simulink model "modelo_lqr_n_linear"  (R2023a)
settings: Solver=ode45  StartTime=0.0  StopTime=10  MaxStep=0.01  RelTol=1e-3
model workspace: external: MATLAB File C:\Users\pinki\OneDrive\aviãozinho\monociclo\numvars.m (data not in the file)
values from neighbouring files (symbols this model uses):
  Ard = [Ar(1,1) Ar(1,3:end) ... (first row only)    [Modelo_mono.m]    (also in workspace.mat = [0 0 -31.2551437046 31.2551437046 0 0 0 0 0 0 -92.3888975157)
  Brd = [Br(1,:) ... (first row only)    [Modelo_mono.m]    (also in workspace.mat = [0  0; 0  0; 50297.8358889  0; -78.116759971  0; 0  238.3657)
  Crd = eye(6)    [Modelo_mono.m]    (also in workspace.mat = [1 0 0 0 0 0 0 1 0 0 0 0 ... (36 elements, 6x6)])
  Jbw = 0.07689    [Modelo_mono.m]    (also in gab_numvars.m; modelo.mat; numvars.m; workspace.mat = 0.026534412)
  Jr = 0.013472    [Modelo_mono.m]    (also in gab_numvars.m; modelo.mat; numvars.m; workspace.mat = 0.0001347355)
  K = lqr(Ard,Brd,Qc,Rc)    [Modelo_mono.m]    (also in cascatinha_v3.m = [tprK,0; workspace.mat = [-891.058429104  -1.00065730536e-12  -0.217264538579  -159.5)
  v_ic = [0;0;0;0]    [Modelo_mono.m]    (also in workspace.mat = [0 0 0 0])
  x_ic = [0;5*pi/180;0;-5*pi/180]    [Modelo_mono.m]    (also in workspace.mat = [0 0.0872664625997 0 -0.0872664625997])
libraries: simulink_extras x1
settings Model: Creator=pinki  LastModifiedBy=pinki
settings DataIOCC: InspectSignalLogs=on

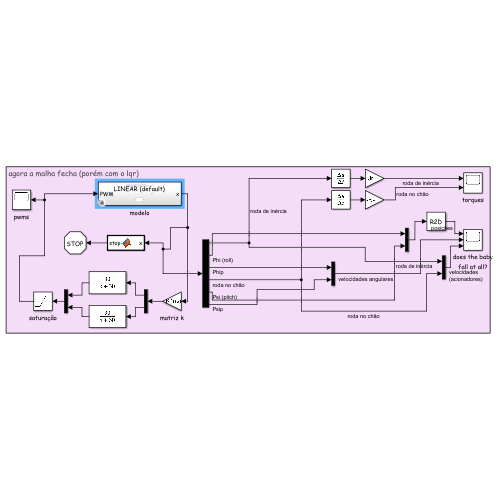
[thumbnail: Simulink's stored preview of the top-level diagram]
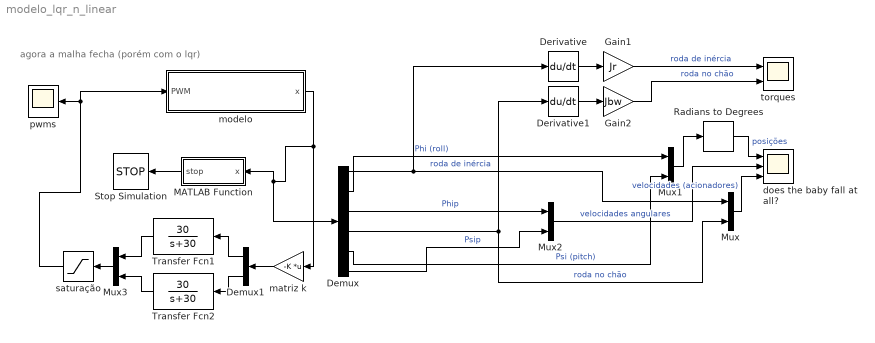
== system modelo_lqr_n_linear ==
  note: agora a malha fecha (porém com o lqr)
  Demux : Demux  Outputs=6
  Demux1 : Demux  Outputs=2
  Derivative : Derivative
  Derivative1 : Derivative
  Gain1 : Gain  Gain=Jr
  Gain2 : Gain  Gain=Jbw
  MATLAB Function : MATLAB Function  TreatAsAtomicUnit=on
  Mux{,1..3} (4 alike) : Mux  Inputs=2
  Radians to Degrees : simulink_extras/Transformations/Radians to Degrees
  Stop Simulation : Stop
  Transfer Fcn1 : TransferFcn  Numerator=[30]  Denominator=[1 30]
  Transfer Fcn2 : TransferFcn  Numerator=[30]  Denominator=[1 30]
  does the baby fall at all? : Scope  NumInputPorts=3
  matriz k : Gain  Gain=-K  Multiplication=Matrix(K*u) (u vector)
  modelo : Subsystem  Variant=on  VariantControlMode=label  LabelModeActiveChoice=(default)
  pwms : Scope
  saturação : Saturate  UpperLimit=1  LowerLimit=-1
  torques : Scope  NumInputPorts=2
  wires:
  modelo/1(x) -> Demux/1, MATLAB Function/1(x), matriz k/1
  Demux/1 -> Derivative/1, Mux/1  "roda de inércia"
  Demux/4 -> Mux/2, Derivative1/1  "roda no chão"
  Demux/3 -> Mux2/1  "Phip"
  saturação/1 -> modelo/1(PWM), pwms/1
  MATLAB Function/1(stop) -> Stop Simulation/1
  Derivative/1 -> Gain1/1
  Gain1/1 -> torques/1  "roda de inércia"
  Derivative1/1 -> Gain2/1
  Gain2/1 -> torques/2  "roda no chão"
  Demux/2 -> Mux1/1  "Phi (roll)"
  Demux/6 -> Mux2/2  "Psip"
  Demux/5 -> Mux1/2  "Psi (pitch)"
  Mux1/1 -> Radians to Degrees/1
  Mux2/1 -> does the baby fall at all?/2  "velocidades angulares"
  Mux/1 -> does the baby fall at all?/3  "velocidades (acionadores)"
  matriz k/1 -> Demux1/1
  Demux1/1 -> Transfer Fcn1/1
  Demux1/2 -> Transfer Fcn2/1
  Transfer Fcn2/1 -> Mux3/2
  Transfer Fcn1/1 -> Mux3/1
  Mux3/1 -> saturação/1
  Radians to Degrees/1 -> does the baby fall at all?/1  "posições"

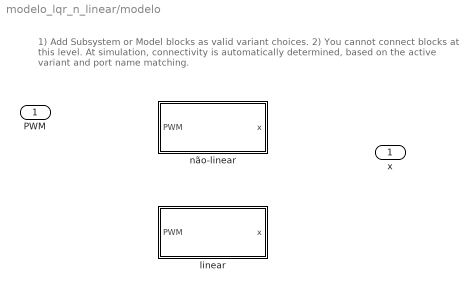
== system modelo_lqr_n_linear/modelo ==
  note: 1) Add Subsystem or Model blocks as valid variant choices.
      | 2) You cannot connect blocks at this level. At simulation, connectivity is automatically
      | determined, based on the active variant and port name matching.
  PWM : Inport
  linear : Subsystem  VariantControl=(default)
  não-linear : Subsystem  VariantControl=nonlinear
  x : Outport

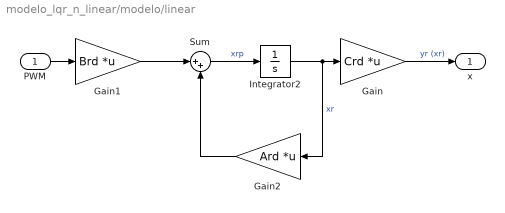
== system modelo_lqr_n_linear/modelo/linear ==
  PWM : Inport
  Gain : Gain  Gain=Crd  Multiplication=Matrix(K*u) (u vector)
  Gain1 : Gain  Gain=Brd  Multiplication=Matrix(K*u) (u vector)
  Gain2 : Gain  Gain=Ard  Multiplication=Matrix(K*u) (u vector)
  Integrator2 : Integrator  InitialCondition=x_ic
  Sum : Sum  Inputs=|++
  x : Outport
  wires:
  PWM/1 -> Gain1/1
  Integrator2/1 -> Gain2/1, Gain/1  "xr"
  Gain/1 -> x/1  "yr (xr)"
  Gain1/1 -> Sum/1
  Sum/1 -> Integrator2/1  "xrp"
  Gain2/1 -> Sum/2

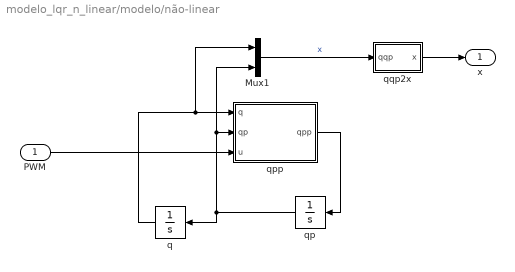
== system modelo_lqr_n_linear/modelo/não-linear ==
  PWM : Inport
  Mux1 : Mux  Inputs=2
  q : Integrator  InitialCondition=x_ic  ContinuousStateAttributes='q'
  qp : Integrator  InitialCondition=v_ic  ContinuousStateAttributes='qp'
  qpp : MATLAB Function  Description=nonlinear model  TreatAsAtomicUnit=on
  qqp2x : Subsystem
  x : Outport
  wires:
  qp/1 -> Mux1/2, qpp/2(qp), q/1
  PWM/1 -> qpp/3(u)
  Mux1/1 -> qqp2x/1(qqp)  "x"
  q/1 -> Mux1/1, qpp/1(q)
  qpp/1(qpp) -> qp/1
  qqp2x/1(x) -> x/1

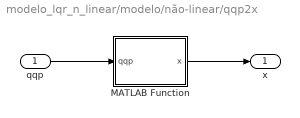
== system modelo_lqr_n_linear/modelo/não-linear/qqp2x ==
  qqp : Inport
  MATLAB Function : MATLAB Function  TreatAsAtomicUnit=on
  x : Outport
  wires:
  qqp/1 -> MATLAB Function/1(qqp)
  MATLAB Function/1(x) -> x/1

== matlab function modelo_lqr_n_linear/MATLAB Function ==
  data: x input; stop output
function stop = fcn(x)

Roll = x(2);
Pitch = x(5);

%% assumindo deslocamento m'aximo de 30 graus ou 0,5 rad...
limite = 0.5;

stop = abs(Pitch)>limite || abs(Roll)>limite;

== matlab function modelo_lqr_n_linear/modelo/não-linear/qqp2x/MATLAB Function ==
  data: qqp input; x output
function x = fcn(qqp)

x = [qqp(5);...
     qqp(2);...
     qqp(6);...
     qqp(7);...
     qqp(4);...
     qqp(8)];

== matlab function modelo_lqr_n_linear/modelo/não-linear/qpp ==
  data: q input; qp input; qpp output; u input
function qpp = fun(q,qp,u)

%% setup
mono = monociclo;

phi = q(2);
psi = q(4);

phi_d = qp(2);
psi_d = qp(4);

thetad_d = qp(1);
thetaw_d = qp(3);

%% setup 2: electric boogaloo
M = fM(mono.jbr, mono.jbw, mono.jr, mono.jw, mono.l, mono.mb, mono.mr, mono.mw, mono.rw, mono.d, psi);
N = fN(mono.ker, mono.kew, mono.ktr, mono.ktw, mono.l, mono.mb, mono.mr, mono.rr, mono.rw, mono.rw, mono.d, mono.nr, mono.nw, phi_d, psi, psi_d, thetad_d, thetaw_d);
O = fO(mono.l, mono.mb, mono.mr, mono.mw, mono.rw, mono.d, mono.g, phi, phi);
P = fP(mono.ktr, mono.ktw, mono.rr, mono.rw, mono.nr, mono.nw);

function M = fM(Jbr,Jbw,Jr,Jw,L,Mb,Mr,Mw,Rw,d,psi_)
%    This function was generated by the Symbolic Math Toolbox version 9.3.

t2 = cos(psi_);
t3 = Mr.*d;
t4 = L.^2;
t5 = Rw.^2;
t7 = L.*Mb;
t8 = L.*Mr;
t9 = t2.^2;
t10 = Mb.*t5;
t11 = Mr.*t5;
t12 = Mw.*t5;
t13 = t3+t7+t8;
t14 = Rw.*t2.*t13;
M = reshape([Jr,Jr,0.0,0.0,Jr,Jbw+Jr+t10+t11+t12+L.*t3.*t9.*2.0+Mb.*t4.*t9+Mr.*t4.*t9+Rw.*t2.*t3.*2.0+Rw.*t2.*t7.*2.0+Rw.*t2.*t8.*2.0+d.*t3.*t9,0.0,0.0,0.0,0.0,Jw+t10+t11+t12,t14,0.0,0.0,t14,Jbr+L.*t3.*2.0+Mb.*t4+Mr.*t4+d.*t3],[4,4]);
end

function N = fN(Ke_d,Ke_w,Kt_d,Kt_w,L,Mb,Mr,R_d,R_w,Rw,d,n_d,n_w,phi_d,psi_,psi_d,thetad_d,thetaw_d)
%    This function was generated by the Symbolic Math Toolbox version 9.3.

t2 = sin(psi_);
t3 = L.^2;
t4 = d.^2;
t5 = n_d.^2;
t6 = n_w.^2;
t7 = phi_d.^2;
t8 = psi_.*2.0;
t9 = psi_d.^2;
t11 = 1.0./R_d;
t12 = 1.0./R_w;
t10 = sin(t8);
t13 = Ke_w.*Kt_w.*n_w.*psi_d.*t12;
t14 = Ke_d.*Kt_d.*t5.*t11.*thetad_d;
t15 = Ke_w.*Kt_w.*t6.*t12.*thetaw_d;
N = [t14;-t14-Mb.*phi_d.*psi_d.*t3.*t10-Mr.*phi_d.*psi_d.*t3.*t10-Mr.*phi_d.*psi_d.*t4.*t10-L.*Mb.*Rw.*phi_d.*psi_d.*t2.*2.0-L.*Mr.*Rw.*phi_d.*psi_d.*t2.*2.0-L.*Mr.*d.*phi_d.*psi_d.*t10.*2.0-Mr.*Rw.*d.*phi_d.*psi_d.*t2.*2.0;-t13+t15-L.*Mb.*Rw.*t2.*t9-L.*Mr.*Rw.*t2.*t9-Mr.*Rw.*d.*t2.*t9;t13-t15+(Mb.*t3.*t7.*t10)./2.0+(Mr.*t3.*t7.*t10)./2.0+(Mr.*t4.*t7.*t10)./2.0+L.*Mb.*Rw.*t2.*t7+L.*Mr.*Rw.*t2.*t7+L.*Mr.*d.*t7.*t10+Mr.*Rw.*d.*t2.*t7];
end

function O = fO(L,Mb,Mr,Mw,Rw,d,g,phi_,psi_)
%    This function was generated by the Symbolic Math Toolbox version 9.3.

t2 = cos(psi_);
O = [0.0;-g.*sin(phi_).*(Mb.*Rw+Mr.*Rw+Mw.*Rw+L.*Mb.*t2+L.*Mr.*t2+Mr.*d.*t2);0.0;-g.*cos(phi_).*sin(psi_).*(Mr.*d+L.*Mb+L.*Mr)];
end

function P = fP(Kt_d,Kt_w,R_d,R_w,n_d,n_w)
%    This function was generated by the Symbolic Math Toolbox version 9.3.

t2 = 1.0./R_d;
t3 = 1.0./R_w;
t4 = Kt_d.*n_d.*t2.*1.2e+1;
t5 = Kt_w.*n_w.*t3.*1.2e+1;
P = reshape([t4,-t4,0.0,0.0,0.0,0.0,t5,-t5],[4,2]);
end

%% calculates qpp
qpp = M\P*u-N-O;

end

% function qpp= fcn(q,qp,u)
% %% setup
% mono = monociclo;
% 
% thetar = q(1);
% thetarp = qp(1);
% 
% phi = q(2);
% phip = qp(2);
% 
% thetaw = q(3);
% thetawp = qp(3);
% 
% psi = q(4);
% psip = qp(4);
% 
% %% matriz m
% m11 = mono.jr;
% m12 = m11;
% m21 = m11;
% m22 = mono.jbw+mono.jr+(mono.mb+mono.mr+mono.mw)*mono.rw^2 ...
% +2*mono.rw*cos(psi)*(mono.l*(mono.mb+mono.mr)+mono.mr*mono.d)...
% +(mono.l^2*(mono.mb+mono.mr)+mono.mr*mono.d^2+2*mono.l*mono.mr*mono.d)*cos(psi)^2;
% m33 = mono.jw+(mono.mb+mono.mr+mono.mw)*mono.rw^2;
% m34 = mono.rw*cos(psi)*(mono.mr*mono.d+mono.l*mono.mb+mono.l*mono.mr);
% m43 = m34;
% m44 = mono.jbr+mono.mb*mono.l^2+mono.mr*mono.l^2+mono.mr*mono.d^2 ...
%     +2*mono.l*mono.mr*mono.d;
% 
% M = zeros(4,4);
%     M(1,1) = m11;
%     M(1,2) = m12;
%     M(2,1) = m21;
%     M(2,2) = m22;
%     M(3,3) = m33;
%     M(3,4) = m34;
%     M(4,3) = m43;
%     M(4,4) = m44;
% 
% %% matriz v
% v1 = (mono.ker*mono.ktr*mono.nr*(mono.nr*thetarp))/mono.rer ...
%      - mono.bvr*thetar;
% v2 = -(mono.ker*mono.ktr*mono.nr*(mono.nr*thetarp))/mono.rer ...
%      - 2*(mono.l*mono.mb+mono.mr*mono.d)*mono.rw*phip*psip*sin(psi) ...
%      - (mono.mr*mono.l^2+mono.mb*mono.l^2+mono.mr*mono.d^2+2*mono.l*mono.mr*mono.d)*phip*psip*sin(2*psi) ...
%      - mono.bvr*thetar;
% v3 = (mono.ker*mono.ktw*mono.nw*(mono.nw*thetawp-psip))/mono.rew ...
%     + (mono.l*mono.mb+mono.d*mono.mr+mono.l*mono.mr)*mono.rw*psip^2*sin(psi) ...
%     + mono.bvw*thetaw;
% v4 = -(mono.ker*mono.ktw*mono.nw*(mono.nw*thetawp-psip))/mono.rew ...
%     + (mono.l*mono.mb+mono.d*mono.mr+mono.l*mono.mr)*mono.rw*phip^2*sin(psi) ...
%     + (sin(2*psi)*phip^2*((mono.mb*mono.l^2)+(mono.mr*mono.l^2) ...
%     + (mono.mr*mono.d^2))/2+mono.l*mono.mr*mono.d)+mono.bvw*thetaw;
% 
% V = zeros(4,1);
%     V(1) = v1;
%     V(2) = v2;
%     V(3) = v3;
%     V(4) = v4;
% 
% %% matriz g
% g2 = -mono.g*sin(phi)*((mono.mb+mono.mr+mono.mw)*mono.rw+(mono.l*mono.mb ...
%     + mono.l*mono.mr + mono.mr*mono.d)*cos(psi));
% g4 = -mono.g*cos(phi)*sin(psi)*(mono.mr*mono.d+mono.l*mono.mb+mono.l*mono.mr);
% 
% G = zeros(4,1);
%     G(2) = g2;
%     G(4) = g4;
% 
% %% matriz p
% p11 = (12*mono.ktr*mono.nr)/mono.rr;
% p12 = -p11;
% p23 = (12*mono.ktw*mono.nw)/mono.rw;
% p24 = -p23;
% 
% P = zeros(4,2);
%     P(1,1) = p11;
%     P(2,1) = p12;
%     P(3,2) = p23;
%     P(4,2) = p24;
% 
% %% qpp
% qpp = M\(-V-G+P*u);
